simulink subsystem "ECEF_coords_to_geodetic"  (R2022a)
settings: Solver=VariableStepAuto  StartTime=0.0  StopTime=10.0  RelTol=1e-3
settings Model: Creator=samuel  LastModifiedBy=samuel

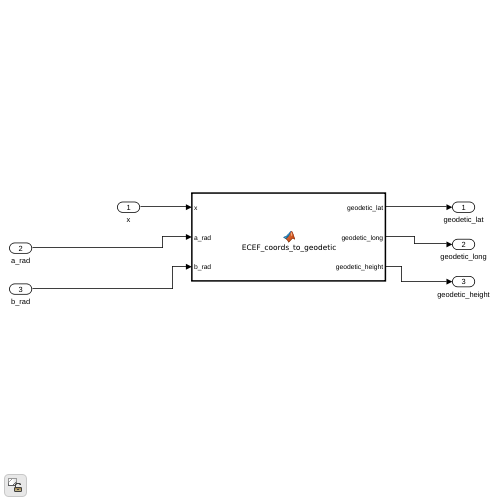
[thumbnail: Simulink's stored preview of the top-level diagram]
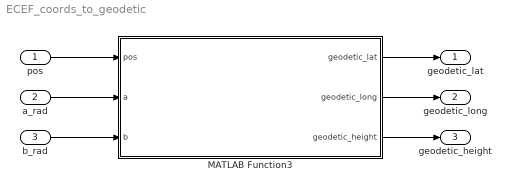
== system ECEF_coords_to_geodetic ==
  pos : Inport
  a_rad : Inport  Port=2
  b_rad : Inport  Port=3
  MATLAB Function3 : MATLAB Function  TreatAsAtomicUnit=on
  geodetic_lat : Outport
  geodetic_long : Outport  Port=2
  geodetic_height : Outport  Port=3
  wires:
  b_rad/1 -> MATLAB Function3/3(b)
  MATLAB Function3/3(geodetic_height) -> geodetic_height/1
  MATLAB Function3/1(geodetic_lat) -> geodetic_lat/1
  MATLAB Function3/2(geodetic_long) -> geodetic_long/1
  pos/1 -> MATLAB Function3/1(pos)
  a_rad/1 -> MATLAB Function3/2(a)

== matlab function ECEF_coords_to_geodetic/MATLAB Function3 ==
  data: pos input; geodetic_lat output; a input; b input; geodetic_long output; geodetic_height output
function [geodetic_lat, geodetic_long, geodetic_height] = ...
    ECEF_coords_to_geodetic(pos, a, b)

    % converts from ECEF coordinates to geodetic coordinates

    x = pos(1);
    y = pos(2);
    z = pos(3);

    e2 = 1 - b^2 / a^2;
    eps2 = a^2 / b^2 - 1;
    rho = sqrt(x^2 + y^2);

    p = abs(z)/eps2;
    s = rho^2/(e2*eps2);
    q = p^2 - b^2 + s;

    u = p/sqrt(q);
    v = b^2*u^2/q;
    P=27*v*s/q;
    Q=(sqrt(P+1) + sqrt(P))^(2/3);

    t=(1+Q+1/Q)/6;
    c=sqrt(u^2-1+2*t);
    w=(c-u)/2;

    d=sign(z)*sqrt(q)*(w+sqrt(t^2+v)-u*w-t/2-1/4);

    N = a*sqrt(1+eps2*d^2/b^2);
    lat = asin((eps2+1)*(d/N));
    
    h = rho*cos(lat)+z*sin(lat)-a^2/N;
    long = atan2(y, x);

    % converts from rad to deg
    geodetic_lat = rad2deg(lat);
    geodetic_long = rad2deg(long);

    geodetic_height = h;
